simulink model "CH13_1C"  (R2021b)
settings: Solver=ode45  StartTime=0.0  StopTime=0.001  RelTol=1e-3  EnableMultiTasking=on
libraries: dsparch4 x1, commsynccomp2 x1
settings Model: Creator=my2  LastModifiedBy=82102
settings SolverCC: AlgebraicLoopSolver=TrustRegion
settings DataIOCC: LimitDataPoints=on  SaveFormat=Array  SignalLoggingSaveFormat=ModelDataLogs  ReturnWorkspaceOutputs=off
settings OptimizationCC: LifeSpan=inf
settings DebuggingCC: UnderspecifiedInitializationDetection=Classic  MergeDetectMultiDrivingBlocksExec=none  SolverPrmCheckMsg=warning  MultiTaskDSMMsg=warning  MultiTaskCondExecSysMsg=none  FcnCallInpInsideContextMsg=warning  SFUnexpectedBacktrackingDiag=warning  SFNoUnconditionalDefaultTransitionDiag=warning  SFExecutionAtInitializationDiag=none  SFMachineParentedDataDiag=warning  ArithmeticOperatorsInVariantConditions=warning
settings HardwareCC: ProdBitPerPointer=32  ProdBitPerSizeT=32  ProdBitPerPtrDiffT=32  ProdLargestAtomicFloat=None  ProdIntDivRoundTo=Undefined  ProdEndianess=Unspecified  ProdWordSize=32  ProdHWDeviceType=32-bit Generic
settings ModelReferenceCC: PropagateSignalLabelsOutOfModel=off
settings SFSimCC: SimUseLocalCustomCode=off  CustomCodeUndefinedFunction=UseInterfaceOnly
settings RTWCC: RTWUseLocalCustomCode=off
settings CodeAppCC: StateflowObjectComments=on
settings GRTTargetCC: TargetLangStandard=C89/C90 (ANSI)  CombineOutputUpdateFcns=off  GRTInterface=on
settings ConfigComp: CovMetricSettings=dw  CovSaveCumulativeToWorkspaceVar=on  CovSaveSingleToWorkspaceVar=on  CovExternalEMLEnable=off

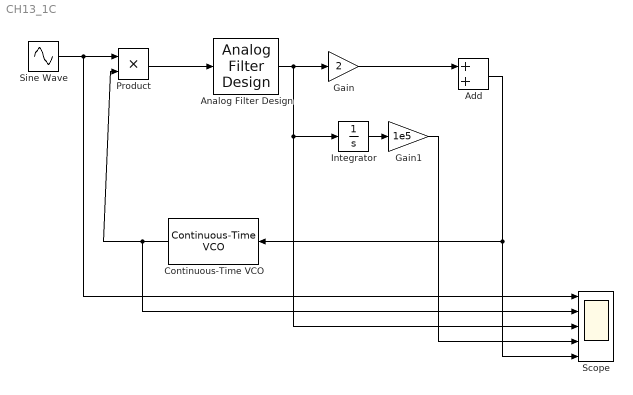
== system CH13_1C ==
  Add : Sum
  Analog Filter Design : dsparch4/Analog Filter Design  method=Chebyshev II  filttype=Lowpass  N=32  Wlo=30  Whi=80  Rp=2  Rs=40
  Continuous-Time VCO : commsynccomp2/Continuous-Time VCO  Ac=1  Fc=93  Kc=1  Ph=0
      settings: SourceProductBaseCode=CM
  Gain : Gain  Gain=2
  Gain1 : Gain  Gain=1e5
  Integrator : Integrator
  Product : Product
  Scope : Scope  NumInputPorts=5
  Sine Wave : Sin  Frequency=94*1000*2*pi  Phase=pi  SampleTime=0
  wires:
  Product/1 -> Analog Filter Design/1
  Analog Filter Design/1 -> Scope/3, Integrator/1, Gain/1
  Integrator/1 -> Gain1/1
  Gain/1 -> Add/1
  Gain1/1 -> Scope/4
  Continuous-Time VCO/1 -> Scope/2, Product/2
  Sine Wave/1 -> Scope/1, Product/1
  Add/1 -> Continuous-Time VCO/1, Scope/5
